simulink model "impedancia"  (R2018a)
settings: Solver=FixedStepAuto  StartTime=0.0  StopTime=20  FixedStep=0.2  RelTol=1e-3
libraries: simulink x1
settings Model: Creator=root  LastModifiedBy=root

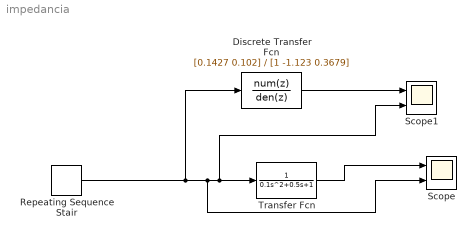
== system impedancia ==
  Discrete Transfer Fcn : DiscreteTransferFcn  Numerator=[0.1427 0.102]  Denominator=[1 -1.123 0.3679]
  Repeating Sequence Stair : simulink/Sources/Repeating Sequence Stair  OutValues=[1 1 1 1 1 1 1 1 1 1 1 1 1 1 ].'  tsamp=-1  OutMin=[]  OutMax=[]  OutDataTypeStr=double  OutputDataTypeScalingMode=double  OutDataType=fixdt(0,8)  ConRadixGroup=Best Precision: Vector-wise  OutScaling=2^-12
  Scope : Scope  NumInputPorts=2
  Scope1 : Scope  NumInputPorts=2
  Transfer Fcn : TransferFcn  Denominator=[0.1 0.5 1]
  wires:
  Repeating Sequence Stair/1 -> Discrete Transfer Fcn/1, Scope1/2, Transfer Fcn/1, Scope/2
  Transfer Fcn/1 -> Scope/1
  Discrete Transfer Fcn/1 -> Scope1/1
